simulink model "ModAMpractica"  (R2019a)
settings: Solver=VariableStepAuto  StartTime=0.0  StopTime=4  RelTol=1e-3
settings Model: Creator=JORGE  LastModifiedBy=JORGE

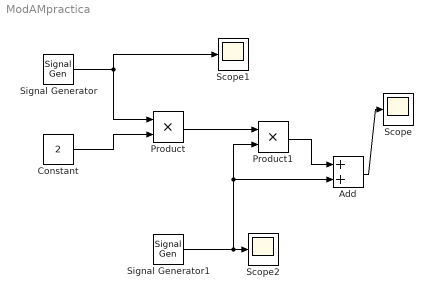
== system ModAMpractica ==
  Add : Sum
  Constant : Constant  Value=2
  Product : Product
  Product1 : Product
  Scope : Scope
  Scope1 : Scope
  Scope2 : Scope
  Signal Generator : SignalGenerator
  Signal Generator1 : SignalGenerator  Frequency=250
  wires:
  Signal Generator/1 -> Scope1/1, Product/1
  Constant/1 -> Product/2
  Product/1 -> Product1/1
  Signal Generator1/1 -> Add/2, Product1/2, Scope2/1
  Product1/1 -> Add/1
  Add/1 -> Scope/1
